simulink library "inp"  (R2021b)
settings: Solver=VariableStepAuto  StartTime=0.0  StopTime=10.0  RelTol=1e-3
undefined symbols (not defined in the file): C_TASK_5MS_S, FALSE, KINP_AcoreReadyToSlp_flg_ovrdflg, KINP_AcoreReadyToSlp_flg_ovrdval, KINP_AllowMovThd_OTA_enum_ovrdflg, KINP_AllowMovThd_OTA_enum_ovrdval, KINP_APSAngleTarget_Deg_ovrdflg, KINP_APSAngleTarget_Deg_ovrdval, KINP_APSDecReq_mps2_ovrdflg, KINP_APSDecReq_mps2_ovrdval, KINP_APSDecReqA_flg_ovrdflg, KINP_APSDecReqA_flg_ovrdval, KINP_APSDFLL_cm_ovrdflg, KINP_APSDFLL_cm_ovrdval, KINP_APSDFLR_cm_ovrdflg, KINP_APSDFLR_cm_ovrdval, KINP_APSDRLL_cm_ovrdflg, KINP_APSDRLL_cm_ovrdval, KINP_APSDRLR_cm_ovrdflg, KINP_APSDRLR_cm_ovrdval, KINP_APSExitCondition_enum_ovrdflg, KINP_APSExitCondition_enum_ovrdval, KINP_APSHWVer_enum_ovrdflg, KINP_APSHWVer_enum_ovrdval, KINP_APSProgressPCT_pct_ovrdflg, KINP_APSProgressPCT_pct_ovrdval, KINP_APSPwrReq_enum_ovrdflg, KINP_APSPwrReq_enum_ovrdval, KINP_APSReq_enum_ovrdflg, KINP_APSReq_enum_ovrdval, KINP_APSRQDisplay_enum_ovrdflg, KINP_APSRQDisplay_enum_ovrdval, KINP_APSRqEPASCtrl_flg_ovrdflg, KINP_APSRqEPASCtrl_flg_ovrdval, KINP_APSShiftPosnReq_enum_ovrdval, KINP_APSShiftPosnReq_enum_ovrflg, KINP_APSSpeedCMD_kph_ovrdval, KINP_APSSpeedCMD_kph_ovrflg, KINP_APSStaSystem_enum_ovrdflg, KINP_APSStaSystem_enum_ovrdval, KINP_APSSWVer_enum_ovrdflg, KINP_APSSWVer_enum_ovrdval, KINP_APSVMCReqA_flg_ovrdval, KINP_APSVMCReqA_flg_ovrflg, KINP_APSVRqEPASCtrl_flg_ovrdflg, KINP_APSVRqEPASCtrl_flg_ovrdval, KINP_AuxBattVolmV_mV_ovrdflg, KINP_AuxBattVolmV_mV_ovrdval, KINP_BTConnectSta_enum_ovrdflg, KINP_BTConnectSta_enum_ovrdval, KINP_CAASSta_enum_ovrdflg, KINP_CAASSta_enum_ovrdval, KINP_CAASVMCReqA_flg_ovrdval, KINP_CAASVMCReqA_flg_ovrflg, KINP_CAN1BusOff_flg_ovrdflg, KINP_CAN1BusOff_flg_ovrdval, KINP_CAN2BusOff_flg_ovrdflg, KINP_CAN2BusOff_flg_ovrdval, KINP_CAN3BusOff_flg_ovrdflg, KINP_CAN3BusOff_flg_ovrdval ... (+222)
libraries: FVT_lib x1035, hcu_lib x1
(part 33 of 33)

== system inp/INP/CAN6/SignalCheck/FCM2 ==
  BHAL_outputs : Inport
  inp_CanValid_bus : Inport  Port=2
  ADBVehDst1Val : FVT_lib/inp/can_signal_template  SystemSampleTime=-1  VariantActivationTime=update diagram  Latency=0  AutoFrameSizeCalculation=off
      link override defval: Value=KINP_ADBVehDst1Val_enum_defval
      link override ovrdflg: Value=KINP_ADBVehDst1Val_enum_ovrdflg
      link override ovrdval: Value=KINP_ADBVehDst1Val_enum_ovrdval
  FCM2CSErr : FVT_lib/inp/can_signal_template  SystemSampleTime=-1  VariantActivationTime=update diagram  Latency=0  AutoFrameSizeCalculation=off
      link override defval: Value=KINP_FCM2CSErr_flg_defval
      link override ovrdflg: Value=KINP_FCM2CSErr_flg_ovrdflg
      link override ovrdval: Value=KINP_FCM2CSErr_flg_ovrdval
  FCM2RCErr : FVT_lib/inp/can_signal_template  SystemSampleTime=-1  VariantActivationTime=update diagram  Latency=0  AutoFrameSizeCalculation=off
      link override defval: Value=KINP_FCM2RCErr_flg_defval
      link override ovrdflg: Value=KINP_FCM2RCErr_flg_ovrdflg
      link override ovrdval: Value=KINP_FCM2RCErr_flg_ovrdval
  Terminator_1 : Terminator
  Terminator_2 : Terminator
  Terminator_3 : Terminator
  True_VHAL_ADBVehDst1Val_enum : Constant  Value=TRUE  OutDataTypeStr=boolean
  True_VHAL_FCM2CSErr_flg : Constant  Value=TRUE  OutDataTypeStr=boolean
  True_VHAL_FCM2RCErr_flg : Constant  Value=TRUE  OutDataTypeStr=boolean
  slr1_1 : BusSelector  OutputSignals=VINP_CANMsgValidFCM2_flg
  slr1_2 : BusSelector  OutputSignals=VINP_CANMsgValidFCM2_flg
  slr1_3 : BusSelector  OutputSignals=VINP_CANMsgValidFCM2_flg
  slr_VHAL_ADBVehDst1Val_enum : BusSelector  OutputSignals=VHAL_ADBVehDst1Val_enum
  slr_VHAL_FCM2CSErr_flg : BusSelector  OutputSignals=VHAL_FCM2CSErr_flg
  slr_VHAL_FCM2RCErr_flg : BusSelector  OutputSignals=VHAL_FCM2RCErr_flg
  VINP_FCM2CSErr_flg : Outport
  VINP_FCM2RCErr_flg : Outport  Port=2
  VINP_ADBVehDst1Val_enum : Outport  Port=3
  wires:
  BHAL_outputs/1 -> [BHAL_outputs]
  inp_CanValid_bus/1 -> [inp_CanValid_bus]
  [BHAL_outputs] -> slr_VHAL_FCM2CSErr_flg/1
  slr_VHAL_FCM2CSErr_flg/1 -> FCM2CSErr/1  "<VHAL_FCM2CSErr_flg>"
  True_VHAL_FCM2CSErr_flg/1 -> FCM2CSErr/2
  [inp_CanValid_bus] -> slr1_1/1
  slr1_1/1 -> FCM2CSErr/3  "<VINP_CANMsgValidFCM2_flg>"
  FCM2CSErr/1 -> VINP_FCM2CSErr_flg/1  "VINP_FCM2CSErr_flg"
  FCM2CSErr/2 -> Terminator_1/1
  [BHAL_outputs] -> slr_VHAL_FCM2RCErr_flg/1
  slr_VHAL_FCM2RCErr_flg/1 -> FCM2RCErr/1  "<VHAL_FCM2RCErr_flg>"
  True_VHAL_FCM2RCErr_flg/1 -> FCM2RCErr/2
  [inp_CanValid_bus] -> slr1_2/1
  slr1_2/1 -> FCM2RCErr/3  "<VINP_CANMsgValidFCM2_flg>"
  FCM2RCErr/1 -> VINP_FCM2RCErr_flg/1  "VINP_FCM2RCErr_flg"
  FCM2RCErr/2 -> Terminator_2/1
  [BHAL_outputs] -> slr_VHAL_ADBVehDst1Val_enum/1
  slr_VHAL_ADBVehDst1Val_enum/1 -> ADBVehDst1Val/1  "<VHAL_ADBVehDst1Val_enum>"
  True_VHAL_ADBVehDst1Val_enum/1 -> ADBVehDst1Val/2
  [inp_CanValid_bus] -> slr1_3/1
  slr1_3/1 -> ADBVehDst1Val/3  "<VINP_CANMsgValidFCM2_flg>"
  ADBVehDst1Val/1 -> VINP_ADBVehDst1Val_enum/1  "VINP_ADBVehDst1Val_enum"
  ADBVehDst1Val/2 -> Terminator_3/1

== system inp/INP/CAN6/SignalCheck/FCM3 ==
  BHAL_outputs : Inport
  inp_CanValid_bus : Inport  Port=2
  MELaneCurvDervLt : FVT_lib/inp/can_signal_template  SystemSampleTime=-1  VariantActivationTime=update diagram  Latency=0  AutoFrameSizeCalculation=off
      link override defval: Value=KINP_MELaneCurvDervLt_raw32_defval
      link override ovrdflg: Value=KINP_MELaneCurvDervLt_raw32_ovrdflg
      link override ovrdval: Value=KINP_MELaneCurvDervLt_raw32_ovrdval
  MELaneCurvDervLt2 : FVT_lib/inp/can_signal_template  SystemSampleTime=-1  VariantActivationTime=update diagram  Latency=0  AutoFrameSizeCalculation=off
      link override defval: Value=KINP_MELaneCurvDervLt2_raw32_defval
      link override ovrdflg: Value=KINP_MELaneCurvDervLt2_raw32_ovrdflg
      link override ovrdval: Value=KINP_MELaneCurvDervLt2_raw32_ovrdval
  MELaneCurvDervRt : FVT_lib/inp/can_signal_template  SystemSampleTime=-1  VariantActivationTime=update diagram  Latency=0  AutoFrameSizeCalculation=off
      link override defval: Value=KINP_MELaneCurvDervRt_raw32_defval
      link override ovrdflg: Value=KINP_MELaneCurvDervRt_raw32_ovrdflg
      link override ovrdval: Value=KINP_MELaneCurvDervRt_raw32_ovrdval
  MELaneCurvDervRt2 : FVT_lib/inp/can_signal_template  SystemSampleTime=-1  VariantActivationTime=update diagram  Latency=0  AutoFrameSizeCalculation=off
      link override defval: Value=KINP_MELaneCurvDervRt2_raw32_defval
      link override ovrdflg: Value=KINP_MELaneCurvDervRt2_raw32_ovrdflg
      link override ovrdval: Value=KINP_MELaneCurvDervRt2_raw32_ovrdval
  MELaneCurvLt : FVT_lib/inp/can_signal_template  SystemSampleTime=-1  VariantActivationTime=update diagram  Latency=0  AutoFrameSizeCalculation=off
      link override defval: Value=KINP_MELaneCurvLt_raw32_defval
      link override ovrdflg: Value=KINP_MELaneCurvLt_raw32_ovrdflg
      link override ovrdval: Value=KINP_MELaneCurvLt_raw32_ovrdval
  MELaneCurvLt2 : FVT_lib/inp/can_signal_template  SystemSampleTime=-1  VariantActivationTime=update diagram  Latency=0  AutoFrameSizeCalculation=off
      link override defval: Value=KINP_MELaneCurvLt2_raw32_defval
      link override ovrdflg: Value=KINP_MELaneCurvLt2_raw32_ovrdflg
      link override ovrdval: Value=KINP_MELaneCurvLt2_raw32_ovrdval
  MELaneCurvRt : FVT_lib/inp/can_signal_template  SystemSampleTime=-1  VariantActivationTime=update diagram  Latency=0  AutoFrameSizeCalculation=off
      link override defval: Value=KINP_MELaneCurvRt_raw32_defval
      link override ovrdflg: Value=KINP_MELaneCurvRt_raw32_ovrdflg
      link override ovrdval: Value=KINP_MELaneCurvRt_raw32_ovrdval
  MELaneCurvRt2 : FVT_lib/inp/can_signal_template  SystemSampleTime=-1  VariantActivationTime=update diagram  Latency=0  AutoFrameSizeCalculation=off
      link override defval: Value=KINP_MELaneCurvRt2_raw32_defval
      link override ovrdflg: Value=KINP_MELaneCurvRt2_raw32_ovrdflg
      link override ovrdval: Value=KINP_MELaneCurvRt2_raw32_ovrdval
  MELaneHeadAngLt : FVT_lib/inp/can_signal_template  SystemSampleTime=-1  VariantActivationTime=update diagram  Latency=0  AutoFrameSizeCalculation=off
      link override defval: Value=KINP_MELaneHeadAngLt_radians_defval
      link override ovrdflg: Value=KINP_MELaneHeadAngLt_radians_ovrdflg
      link override ovrdval: Value=KINP_MELaneHeadAngLt_radians_ovrdval
  MELaneHeadAngLt2 : FVT_lib/inp/can_signal_template  SystemSampleTime=-1  VariantActivationTime=update diagram  Latency=0  AutoFrameSizeCalculation=off
      link override defval: Value=KINP_MELaneHeadAngLt2_radians_defval
      link override ovrdflg: Value=KINP_MELaneHeadAngLt2_radians_ovrdflg
      link override ovrdval: Value=KINP_MELaneHeadAngLt2_radians_ovrdval
  MELaneHeadAngRt : FVT_lib/inp/can_signal_template  SystemSampleTime=-1  VariantActivationTime=update diagram  Latency=0  AutoFrameSizeCalculation=off
      link override defval: Value=KINP_MELaneHeadAngRt_radians_defval
      link override ovrdflg: Value=KINP_MELaneHeadAngRt_radians_ovrdflg
      link override ovrdval: Value=KINP_MELaneHeadAngRt_radians_ovrdval
  MELaneHeadAngRt2 : FVT_lib/inp/can_signal_template  SystemSampleTime=-1  VariantActivationTime=update diagram  Latency=0  AutoFrameSizeCalculation=off
      link override defval: Value=KINP_MELaneHeadAngRt2_radians_defval
      link override ovrdflg: Value=KINP_MELaneHeadAngRt2_radians_ovrdflg
      link override ovrdval: Value=KINP_MELaneHeadAngRt2_radians_ovrdval
  MELanePosLt : FVT_lib/inp/can_signal_template  SystemSampleTime=-1  VariantActivationTime=update diagram  Latency=0  AutoFrameSizeCalculation=off
      link override defval: Value=KINP_MELanePosLt_m_defval
      link override ovrdflg: Value=KINP_MELanePosLt_m_ovrdflg
      link override ovrdval: Value=KINP_MELanePosLt_m_ovrdval
  MELanePosLt2 : FVT_lib/inp/can_signal_template  SystemSampleTime=-1  VariantActivationTime=update diagram  Latency=0  AutoFrameSizeCalculation=off
      link override defval: Value=KINP_MELanePosLt2_m_defval
      link override ovrdflg: Value=KINP_MELanePosLt2_m_ovrdflg
      link override ovrdval: Value=KINP_MELanePosLt2_m_ovrdval
  MELanePosRt : FVT_lib/inp/can_signal_template  SystemSampleTime=-1  VariantActivationTime=update diagram  Latency=0  AutoFrameSizeCalculation=off
      link override defval: Value=KINP_MELanePosRt_m_defval
      link override ovrdflg: Value=KINP_MELanePosRt_m_ovrdflg
      link override ovrdval: Value=KINP_MELanePosRt_m_ovrdval
  MELanePosRt2 : FVT_lib/inp/can_signal_template  SystemSampleTime=-1  VariantActivationTime=update diagram  Latency=0  AutoFrameSizeCalculation=off
      link override defval: Value=KINP_MELanePosRt2_m_defval
      link override ovrdflg: Value=KINP_MELanePosRt2_m_ovrdflg
      link override ovrdval: Value=KINP_MELanePosRt2_m_ovrdval
  Terminator_{1..16} (16 alike) : Terminator
  True_VHAL_MELaneCurvDervLt2_raw32 : Constant  Value=TRUE  OutDataTypeStr=boolean
  True_VHAL_MELaneCurvDervLt_raw32 : Constant  Value=TRUE  OutDataTypeStr=boolean
  True_VHAL_MELaneCurvDervRt2_raw32 : Constant  Value=TRUE  OutDataTypeStr=boolean
  True_VHAL_MELaneCurvDervRt_raw32 : Constant  Value=TRUE  OutDataTypeStr=boolean
  True_VHAL_MELaneCurvLt2_raw32 : Constant  Value=TRUE  OutDataTypeStr=boolean
  True_VHAL_MELaneCurvLt_raw32 : Constant  Value=TRUE  OutDataTypeStr=boolean
  True_VHAL_MELaneCurvRt2_raw32 : Constant  Value=TRUE  OutDataTypeStr=boolean
  True_VHAL_MELaneCurvRt_raw32 : Constant  Value=TRUE  OutDataTypeStr=boolean
  True_VHAL_MELaneHeadAngLt2_radians : Constant  Value=TRUE  OutDataTypeStr=boolean
  True_VHAL_MELaneHeadAngLt_radians : Constant  Value=TRUE  OutDataTypeStr=boolean
  True_VHAL_MELaneHeadAngRt2_radians : Constant  Value=TRUE  OutDataTypeStr=boolean
  True_VHAL_MELaneHeadAngRt_radians : Constant  Value=TRUE  OutDataTypeStr=boolean
  True_VHAL_MELanePosLt2_m : Constant  Value=TRUE  OutDataTypeStr=boolean
  True_VHAL_MELanePosLt_m : Constant  Value=TRUE  OutDataTypeStr=boolean
  True_VHAL_MELanePosRt2_m : Constant  Value=TRUE  OutDataTypeStr=boolean
  True_VHAL_MELanePosRt_m : Constant  Value=TRUE  OutDataTypeStr=boolean
  slr1_{1..16} (16 alike) : BusSelector  OutputSignals=VINP_CANMsgValidFCM3_flg
  slr_VHAL_MELaneCurvDervLt2_raw32 : BusSelector  OutputSignals=VHAL_MELaneCurvDervLt2_raw32
  slr_VHAL_MELaneCurvDervLt_raw32 : BusSelector  OutputSignals=VHAL_MELaneCurvDervLt_raw32
  slr_VHAL_MELaneCurvDervRt2_raw32 : BusSelector  OutputSignals=VHAL_MELaneCurvDervRt2_raw32
  slr_VHAL_MELaneCurvDervRt_raw32 : BusSelector  OutputSignals=VHAL_MELaneCurvDervRt_raw32
  slr_VHAL_MELaneCurvLt2_raw32 : BusSelector  OutputSignals=VHAL_MELaneCurvLt2_raw32
  slr_VHAL_MELaneCurvLt_raw32 : BusSelector  OutputSignals=VHAL_MELaneCurvLt_raw32
  slr_VHAL_MELaneCurvRt2_raw32 : BusSelector  OutputSignals=VHAL_MELaneCurvRt2_raw32
  slr_VHAL_MELaneCurvRt_raw32 : BusSelector  OutputSignals=VHAL_MELaneCurvRt_raw32
  slr_VHAL_MELaneHeadAngLt2_radians : BusSelector  OutputSignals=VHAL_MELaneHeadAngLt2_radians
  slr_VHAL_MELaneHeadAngLt_radians : BusSelector  OutputSignals=VHAL_MELaneHeadAngLt_radians
  slr_VHAL_MELaneHeadAngRt2_radians : BusSelector  OutputSignals=VHAL_MELaneHeadAngRt2_radians
  slr_VHAL_MELaneHeadAngRt_radians : BusSelector  OutputSignals=VHAL_MELaneHeadAngRt_radians
  slr_VHAL_MELanePosLt2_m : BusSelector  OutputSignals=VHAL_MELanePosLt2_m
  slr_VHAL_MELanePosLt_m : BusSelector  OutputSignals=VHAL_MELanePosLt_m
  slr_VHAL_MELanePosRt2_m : BusSelector  OutputSignals=VHAL_MELanePosRt2_m
  slr_VHAL_MELanePosRt_m : BusSelector  OutputSignals=VHAL_MELanePosRt_m
  VINP_MELaneCurvDervLt_raw32 : Outport
  VINP_MELaneCurvDervLt2_raw32 : Outport  Port=2
  VINP_MELaneCurvDervRt_raw32 : Outport  Port=3
  VINP_MELaneCurvDervRt2_raw32 : Outport  Port=4
  VINP_MELaneCurvLt_raw32 : Outport  Port=5
  VINP_MELaneCurvLt2_raw32 : Outport  Port=6
  VINP_MELaneCurvRt_raw32 : Outport  Port=7
  VINP_MELaneCurvRt2_raw32 : Outport  Port=8
  VINP_MELaneHeadAngLt_radians : Outport  Port=9
  VINP_MELaneHeadAngLt2_radians : Outport  Port=10
  VINP_MELaneHeadAngRt_radians : Outport  Port=11
  VINP_MELaneHeadAngRt2_radians : Outport  Port=12
  VINP_MELanePosLt_m : Outport  Port=13
  VINP_MELanePosLt2_m : Outport  Port=14
  VINP_MELanePosRt_m : Outport  Port=15
  VINP_MELanePosRt2_m : Outport  Port=16
  wires:
  BHAL_outputs/1 -> [BHAL_outputs]
  inp_CanValid_bus/1 -> [inp_CanValid_bus]
  [BHAL_outputs] -> slr_VHAL_MELaneCurvDervLt_raw32/1
  slr_VHAL_MELaneCurvDervLt_raw32/1 -> MELaneCurvDervLt/1  "<VHAL_MELaneCurvDervLt_raw32>"
  True_VHAL_MELaneCurvDervLt_raw32/1 -> MELaneCurvDervLt/2
  [inp_CanValid_bus] -> slr1_1/1
  slr1_1/1 -> MELaneCurvDervLt/3  "<VINP_CANMsgValidFCM3_flg>"
  MELaneCurvDervLt/1 -> VINP_MELaneCurvDervLt_raw32/1  "VINP_MELaneCurvDervLt_raw32"
  MELaneCurvDervLt/2 -> Terminator_1/1
  [BHAL_outputs] -> slr_VHAL_MELaneCurvDervLt2_raw32/1
  slr_VHAL_MELaneCurvDervLt2_raw32/1 -> MELaneCurvDervLt2/1  "<VHAL_MELaneCurvDervLt2_raw32>"
  True_VHAL_MELaneCurvDervLt2_raw32/1 -> MELaneCurvDervLt2/2
  [inp_CanValid_bus] -> slr1_2/1
  slr1_2/1 -> MELaneCurvDervLt2/3  "<VINP_CANMsgValidFCM3_flg>"
  MELaneCurvDervLt2/1 -> VINP_MELaneCurvDervLt2_raw32/1  "VINP_MELaneCurvDervLt2_raw32"
  MELaneCurvDervLt2/2 -> Terminator_2/1
  [BHAL_outputs] -> slr_VHAL_MELaneCurvDervRt_raw32/1
  slr_VHAL_MELaneCurvDervRt_raw32/1 -> MELaneCurvDervRt/1  "<VHAL_MELaneCurvDervRt_raw32>"
  True_VHAL_MELaneCurvDervRt_raw32/1 -> MELaneCurvDervRt/2
  [inp_CanValid_bus] -> slr1_3/1
  slr1_3/1 -> MELaneCurvDervRt/3  "<VINP_CANMsgValidFCM3_flg>"
  MELaneCurvDervRt/1 -> VINP_MELaneCurvDervRt_raw32/1  "VINP_MELaneCurvDervRt_raw32"
  MELaneCurvDervRt/2 -> Terminator_3/1
  [BHAL_outputs] -> slr_VHAL_MELaneCurvDervRt2_raw32/1
  slr_VHAL_MELaneCurvDervRt2_raw32/1 -> MELaneCurvDervRt2/1  "<VHAL_MELaneCurvDervRt2_raw32>"
  True_VHAL_MELaneCurvDervRt2_raw32/1 -> MELaneCurvDervRt2/2
  [inp_CanValid_bus] -> slr1_4/1
  slr1_4/1 -> MELaneCurvDervRt2/3  "<VINP_CANMsgValidFCM3_flg>"
  MELaneCurvDervRt2/1 -> VINP_MELaneCurvDervRt2_raw32/1  "VINP_MELaneCurvDervRt2_raw32"
  MELaneCurvDervRt2/2 -> Terminator_4/1
  [BHAL_outputs] -> slr_VHAL_MELaneCurvLt_raw32/1
  slr_VHAL_MELaneCurvLt_raw32/1 -> MELaneCurvLt/1  "<VHAL_MELaneCurvLt_raw32>"
  True_VHAL_MELaneCurvLt_raw32/1 -> MELaneCurvLt/2
  [inp_CanValid_bus] -> slr1_5/1
  slr1_5/1 -> MELaneCurvLt/3  "<VINP_CANMsgValidFCM3_flg>"
  MELaneCurvLt/1 -> VINP_MELaneCurvLt_raw32/1  "VINP_MELaneCurvLt_raw32"
  MELaneCurvLt/2 -> Terminator_5/1
  [BHAL_outputs] -> slr_VHAL_MELaneCurvLt2_raw32/1
  slr_VHAL_MELaneCurvLt2_raw32/1 -> MELaneCurvLt2/1  "<VHAL_MELaneCurvLt2_raw32>"
  True_VHAL_MELaneCurvLt2_raw32/1 -> MELaneCurvLt2/2
  [inp_CanValid_bus] -> slr1_6/1
  slr1_6/1 -> MELaneCurvLt2/3  "<VINP_CANMsgValidFCM3_flg>"
  MELaneCurvLt2/1 -> VINP_MELaneCurvLt2_raw32/1  "VINP_MELaneCurvLt2_raw32"
  MELaneCurvLt2/2 -> Terminator_6/1
  [BHAL_outputs] -> slr_VHAL_MELaneCurvRt_raw32/1
  slr_VHAL_MELaneCurvRt_raw32/1 -> MELaneCurvRt/1  "<VHAL_MELaneCurvRt_raw32>"
  True_VHAL_MELaneCurvRt_raw32/1 -> MELaneCurvRt/2
  [inp_CanValid_bus] -> slr1_7/1
  slr1_7/1 -> MELaneCurvRt/3  "<VINP_CANMsgValidFCM3_flg>"
  MELaneCurvRt/1 -> VINP_MELaneCurvRt_raw32/1  "VINP_MELaneCurvRt_raw32"
  MELaneCurvRt/2 -> Terminator_7/1
  [BHAL_outputs] -> slr_VHAL_MELaneCurvRt2_raw32/1
  slr_VHAL_MELaneCurvRt2_raw32/1 -> MELaneCurvRt2/1  "<VHAL_MELaneCurvRt2_raw32>"
  True_VHAL_MELaneCurvRt2_raw32/1 -> MELaneCurvRt2/2
  [inp_CanValid_bus] -> slr1_8/1
  slr1_8/1 -> MELaneCurvRt2/3  "<VINP_CANMsgValidFCM3_flg>"
  MELaneCurvRt2/1 -> VINP_MELaneCurvRt2_raw32/1  "VINP_MELaneCurvRt2_raw32"
  MELaneCurvRt2/2 -> Terminator_8/1
  [BHAL_outputs] -> slr_VHAL_MELaneHeadAngLt_radians/1
  slr_VHAL_MELaneHeadAngLt_radians/1 -> MELaneHeadAngLt/1  "<VHAL_MELaneHeadAngLt_radians>"
  True_VHAL_MELaneHeadAngLt_radians/1 -> MELaneHeadAngLt/2
  [inp_CanValid_bus] -> slr1_9/1
  slr1_9/1 -> MELaneHeadAngLt/3  "<VINP_CANMsgValidFCM3_flg>"
  MELaneHeadAngLt/1 -> VINP_MELaneHeadAngLt_radians/1  "VINP_MELaneHeadAngLt_radians"
  MELaneHeadAngLt/2 -> Terminator_9/1
  [BHAL_outputs] -> slr_VHAL_MELaneHeadAngLt2_radians/1
  slr_VHAL_MELaneHeadAngLt2_radians/1 -> MELaneHeadAngLt2/1  "<VHAL_MELaneHeadAngLt2_radians>"
  True_VHAL_MELaneHeadAngLt2_radians/1 -> MELaneHeadAngLt2/2
  [inp_CanValid_bus] -> slr1_10/1
  slr1_10/1 -> MELaneHeadAngLt2/3  "<VINP_CANMsgValidFCM3_flg>"
  MELaneHeadAngLt2/1 -> VINP_MELaneHeadAngLt2_radians/1  "VINP_MELaneHeadAngLt2_radians"
  MELaneHeadAngLt2/2 -> Terminator_10/1
  [BHAL_outputs] -> slr_VHAL_MELaneHeadAngRt_radians/1
  slr_VHAL_MELaneHeadAngRt_radians/1 -> MELaneHeadAngRt/1  "<VHAL_MELaneHeadAngRt_radians>"
  True_VHAL_MELaneHeadAngRt_radians/1 -> MELaneHeadAngRt/2
  [inp_CanValid_bus] -> slr1_11/1
  slr1_11/1 -> MELaneHeadAngRt/3  "<VINP_CANMsgValidFCM3_flg>"
  MELaneHeadAngRt/1 -> VINP_MELaneHeadAngRt_radians/1  "VINP_MELaneHeadAngRt_radians"
  MELaneHeadAngRt/2 -> Terminator_11/1
  [BHAL_outputs] -> slr_VHAL_MELaneHeadAngRt2_radians/1
  slr_VHAL_MELaneHeadAngRt2_radians/1 -> MELaneHeadAngRt2/1  "<VHAL_MELaneHeadAngRt2_radians>"
  True_VHAL_MELaneHeadAngRt2_radians/1 -> MELaneHeadAngRt2/2
  [inp_CanValid_bus] -> slr1_12/1
  slr1_12/1 -> MELaneHeadAngRt2/3  "<VINP_CANMsgValidFCM3_flg>"
  MELaneHeadAngRt2/1 -> VINP_MELaneHeadAngRt2_radians/1  "VINP_MELaneHeadAngRt2_radians"
  MELaneHeadAngRt2/2 -> Terminator_12/1
  [BHAL_outputs] -> slr_VHAL_MELanePosLt_m/1
  slr_VHAL_MELanePosLt_m/1 -> MELanePosLt/1  "<VHAL_MELanePosLt_m>"
  True_VHAL_MELanePosLt_m/1 -> MELanePosLt/2
  [inp_CanValid_bus] -> slr1_13/1
  slr1_13/1 -> MELanePosLt/3  "<VINP_CANMsgValidFCM3_flg>"
  MELanePosLt/1 -> VINP_MELanePosLt_m/1  "VINP_MELanePosLt_m"
  MELanePosLt/2 -> Terminator_13/1
  [BHAL_outputs] -> slr_VHAL_MELanePosLt2_m/1
  slr_VHAL_MELanePosLt2_m/1 -> MELanePosLt2/1  "<VHAL_MELanePosLt2_m>"
  True_VHAL_MELanePosLt2_m/1 -> MELanePosLt2/2
  [inp_CanValid_bus] -> slr1_14/1
  slr1_14/1 -> MELanePosLt2/3  "<VINP_CANMsgValidFCM3_flg>"
  MELanePosLt2/1 -> VINP_MELanePosLt2_m/1  "VINP_MELanePosLt2_m"
  MELanePosLt2/2 -> Terminator_14/1
  [BHAL_outputs] -> slr_VHAL_MELanePosRt_m/1
  slr_VHAL_MELanePosRt_m/1 -> MELanePosRt/1  "<VHAL_MELanePosRt_m>"
  True_VHAL_MELanePosRt_m/1 -> MELanePosRt/2
  [inp_CanValid_bus] -> slr1_15/1
  slr1_15/1 -> MELanePosRt/3  "<VINP_CANMsgValidFCM3_flg>"
  MELanePosRt/1 -> VINP_MELanePosRt_m/1  "VINP_MELanePosRt_m"
  MELanePosRt/2 -> Terminator_15/1
  [BHAL_outputs] -> slr_VHAL_MELanePosRt2_m/1
  slr_VHAL_MELanePosRt2_m/1 -> MELanePosRt2/1  "<VHAL_MELanePosRt2_m>"
  True_VHAL_MELanePosRt2_m/1 -> MELanePosRt2/2
  [inp_CanValid_bus] -> slr1_16/1
  slr1_16/1 -> MELanePosRt2/3  "<VINP_CANMsgValidFCM3_flg>"
  MELanePosRt2/1 -> VINP_MELanePosRt2_m/1  "VINP_MELanePosRt2_m"
  MELanePosRt2/2 -> Terminator_16/1

== system inp/INP/CAN6/SignalCheck/FCM4 ==
  BHAL_outputs : Inport
  inp_CanValid_bus : Inport  Port=2
  ADASAngCtrlTqWeightGain : FVT_lib/inp/can_signal_template  SystemSampleTime=-1  VariantActivationTime=update diagram  Latency=0  AutoFrameSizeCalculation=off
      link override defval: Value=KINP_ADASAngCtrlTqWeightGain_pct_defval
      link override ovrdflg: Value=KINP_ADASAngCtrlTqWeightGain_pct_ovrdflg
      link override ovrdval: Value=KINP_ADASAngCtrlTqWeightGain_pct_ovrdval
  ADASDesStrWhlAngCtrlCmd : FVT_lib/inp/can_signal_template  SystemSampleTime=-1  VariantActivationTime=update diagram  Latency=0  AutoFrameSizeCalculation=off
      link override defval: Value=KINP_ADASDesStrWhlAngCtrlCmd_Deg_defval
      link override ovrdflg: Value=KINP_ADASDesStrWhlAngCtrlCmd_Deg_ovrdflg
      link override ovrdval: Value=KINP_ADASDesStrWhlAngCtrlCmd_Deg_ovrdval
  ADASDrvInputTqBoostAct : FVT_lib/inp/can_signal_template  SystemSampleTime=-1  VariantActivationTime=update diagram  Latency=0  AutoFrameSizeCalculation=off
      link override defval: Value=KINP_ADASDrvInputTqBoostAct_flg_defval
      link override ovrdflg: Value=KINP_ADASDrvInputTqBoostAct_flg_ovrdflg
      link override ovrdval: Value=KINP_ADASDrvInputTqBoostAct_flg_ovrdval
  ADASDrvInputTqBoostGain : FVT_lib/inp/can_signal_template  SystemSampleTime=-1  VariantActivationTime=update diagram  Latency=0  AutoFrameSizeCalculation=off
      link override defval: Value=KINP_ADASDrvInputTqBoostGain_pct_defval
      link override ovrdflg: Value=KINP_ADASDrvInputTqBoostGain_pct_ovrdflg
      link override ovrdval: Value=KINP_ADASDrvInputTqBoostGain_pct_ovrdval
  ADASMaxAngCtrlOutTqLimit : FVT_lib/inp/can_signal_template  SystemSampleTime=-1  VariantActivationTime=update diagram  Latency=0  AutoFrameSizeCalculation=off
      link override defval: Value=KINP_ADASMaxAngCtrlOutTqLimit_Nm_defval
      link override ovrdflg: Value=KINP_ADASMaxAngCtrlOutTqLimit_Nm_ovrdflg
      link override ovrdval: Value=KINP_ADASMaxAngCtrlOutTqLimit_Nm_ovrdval
  ADASStrWhlAngCtrlStatus : FVT_lib/inp/can_signal_template  SystemSampleTime=-1  VariantActivationTime=update diagram  Latency=0  AutoFrameSizeCalculation=off
      link override defval: Value=KINP_ADASStrWhlAngCtrlStatus_flg_defval
      link override ovrdflg: Value=KINP_ADASStrWhlAngCtrlStatus_flg_ovrdflg
      link override ovrdval: Value=KINP_ADASStrWhlAngCtrlStatus_flg_ovrdval
  FCM4CSErr : FVT_lib/inp/can_signal_template  SystemSampleTime=-1  VariantActivationTime=update diagram  Latency=0  AutoFrameSizeCalculation=off
      link override defval: Value=KINP_FCM4CSErr_flg_defval
      link override ovrdflg: Value=KINP_FCM4CSErr_flg_ovrdflg
      link override ovrdval: Value=KINP_FCM4CSErr_flg_ovrdval
  FCM4RCErr : FVT_lib/inp/can_signal_template  SystemSampleTime=-1  VariantActivationTime=update diagram  Latency=0  AutoFrameSizeCalculation=off
      link override defval: Value=KINP_FCM4RCErr_flg_defval
      link override ovrdflg: Value=KINP_FCM4RCErr_flg_ovrdflg
      link override ovrdval: Value=KINP_FCM4RCErr_flg_ovrdval
  Terminator_{1..8} (8 alike) : Terminator
  True_VHAL_ADASAngCtrlTqWeightGain_pct : Constant  Value=TRUE  OutDataTypeStr=boolean
  True_VHAL_ADASDesStrWhlAngCtrlCmd_Deg : Constant  Value=TRUE  OutDataTypeStr=boolean
  True_VHAL_ADASDrvInputTqBoostAct_flg : Constant  Value=TRUE  OutDataTypeStr=boolean
  True_VHAL_ADASDrvInputTqBoostGain_pct : Constant  Value=TRUE  OutDataTypeStr=boolean
  True_VHAL_ADASMaxAngCtrlOutTqLimit_Nm : Constant  Value=TRUE  OutDataTypeStr=boolean
  True_VHAL_ADASStrWhlAngCtrlStatus_flg : Constant  Value=TRUE  OutDataTypeStr=boolean
  True_VHAL_FCM4CSErr_flg : Constant  Value=TRUE  OutDataTypeStr=boolean
  True_VHAL_FCM4RCErr_flg : Constant  Value=TRUE  OutDataTypeStr=boolean
  slr1_{1..8} (8 alike) : BusSelector  OutputSignals=VINP_CANMsgValidFCM4_flg
  slr_VHAL_ADASAngCtrlTqWeightGain_pct : BusSelector  OutputSignals=VHAL_ADASAngCtrlTqWeightGain_pct
  slr_VHAL_ADASDesStrWhlAngCtrlCmd_Deg : BusSelector  OutputSignals=VHAL_ADASDesStrWhlAngCtrlCmd_Deg
  slr_VHAL_ADASDrvInputTqBoostAct_flg : BusSelector  OutputSignals=VHAL_ADASDrvInputTqBoostAct_flg
  slr_VHAL_ADASDrvInputTqBoostGain_pct : BusSelector  OutputSignals=VHAL_ADASDrvInputTqBoostGain_pct
  slr_VHAL_ADASMaxAngCtrlOutTqLimit_Nm : BusSelector  OutputSignals=VHAL_ADASMaxAngCtrlOutTqLimit_Nm
  slr_VHAL_ADASStrWhlAngCtrlStatus_flg : BusSelector  OutputSignals=VHAL_ADASStrWhlAngCtrlStatus_flg
  slr_VHAL_FCM4CSErr_flg : BusSelector  OutputSignals=VHAL_FCM4CSErr_flg
  slr_VHAL_FCM4RCErr_flg : BusSelector  OutputSignals=VHAL_FCM4RCErr_flg
  VINP_FCM4CSErr_flg : Outport
  VINP_FCM4RCErr_flg : Outport  Port=2
  VINP_ADASAngCtrlTqWeightGain_pct : Outport  Port=3
  VINP_ADASDesStrWhlAngCtrlCmd_Deg : Outport  Port=4
  VINP_ADASDrvInputTqBoostAct_flg : Outport  Port=5
  VINP_ADASDrvInputTqBoostGain_pct : Outport  Port=6
  VINP_ADASMaxAngCtrlOutTqLimit_Nm : Outport  Port=7
  VINP_ADASStrWhlAngCtrlStatus_flg : Outport  Port=8
  wires:
  BHAL_outputs/1 -> [BHAL_outputs]
  inp_CanValid_bus/1 -> [inp_CanValid_bus]
  [BHAL_outputs] -> slr_VHAL_FCM4CSErr_flg/1
  slr_VHAL_FCM4CSErr_flg/1 -> FCM4CSErr/1  "<VHAL_FCM4CSErr_flg>"
  True_VHAL_FCM4CSErr_flg/1 -> FCM4CSErr/2
  [inp_CanValid_bus] -> slr1_1/1
  slr1_1/1 -> FCM4CSErr/3  "<VINP_CANMsgValidFCM4_flg>"
  FCM4CSErr/1 -> VINP_FCM4CSErr_flg/1  "VINP_FCM4CSErr_flg"
  FCM4CSErr/2 -> Terminator_1/1
  [BHAL_outputs] -> slr_VHAL_FCM4RCErr_flg/1
  slr_VHAL_FCM4RCErr_flg/1 -> FCM4RCErr/1  "<VHAL_FCM4RCErr_flg>"
  True_VHAL_FCM4RCErr_flg/1 -> FCM4RCErr/2
  [inp_CanValid_bus] -> slr1_2/1
  slr1_2/1 -> FCM4RCErr/3  "<VINP_CANMsgValidFCM4_flg>"
  FCM4RCErr/1 -> VINP_FCM4RCErr_flg/1  "VINP_FCM4RCErr_flg"
  FCM4RCErr/2 -> Terminator_2/1
  [BHAL_outputs] -> slr_VHAL_ADASAngCtrlTqWeightGain_pct/1
  slr_VHAL_ADASAngCtrlTqWeightGain_pct/1 -> ADASAngCtrlTqWeightGain/1  "<VHAL_ADASAngCtrlTqWeightGain_pct>"
  True_VHAL_ADASAngCtrlTqWeightGain_pct/1 -> ADASAngCtrlTqWeightGain/2
  [inp_CanValid_bus] -> slr1_3/1
  slr1_3/1 -> ADASAngCtrlTqWeightGain/3  "<VINP_CANMsgValidFCM4_flg>"
  ADASAngCtrlTqWeightGain/1 -> VINP_ADASAngCtrlTqWeightGain_pct/1  "VINP_ADASAngCtrlTqWeightGain_pct"
  ADASAngCtrlTqWeightGain/2 -> Terminator_3/1
  [BHAL_outputs] -> slr_VHAL_ADASDesStrWhlAngCtrlCmd_Deg/1
  slr_VHAL_ADASDesStrWhlAngCtrlCmd_Deg/1 -> ADASDesStrWhlAngCtrlCmd/1  "<VHAL_ADASDesStrWhlAngCtrlCmd_Deg>"
  True_VHAL_ADASDesStrWhlAngCtrlCmd_Deg/1 -> ADASDesStrWhlAngCtrlCmd/2
  [inp_CanValid_bus] -> slr1_4/1
  slr1_4/1 -> ADASDesStrWhlAngCtrlCmd/3  "<VINP_CANMsgValidFCM4_flg>"
  ADASDesStrWhlAngCtrlCmd/1 -> VINP_ADASDesStrWhlAngCtrlCmd_Deg/1  "VINP_ADASDesStrWhlAngCtrlCmd_Deg"
  ADASDesStrWhlAngCtrlCmd/2 -> Terminator_4/1
  [BHAL_outputs] -> slr_VHAL_ADASDrvInputTqBoostAct_flg/1
  slr_VHAL_ADASDrvInputTqBoostAct_flg/1 -> ADASDrvInputTqBoostAct/1  "<VHAL_ADASDrvInputTqBoostAct_flg>"
  True_VHAL_ADASDrvInputTqBoostAct_flg/1 -> ADASDrvInputTqBoostAct/2
  [inp_CanValid_bus] -> slr1_5/1
  slr1_5/1 -> ADASDrvInputTqBoostAct/3  "<VINP_CANMsgValidFCM4_flg>"
  ADASDrvInputTqBoostAct/1 -> VINP_ADASDrvInputTqBoostAct_flg/1  "VINP_ADASDrvInputTqBoostAct_flg"
  ADASDrvInputTqBoostAct/2 -> Terminator_5/1
  [BHAL_outputs] -> slr_VHAL_ADASDrvInputTqBoostGain_pct/1
  slr_VHAL_ADASDrvInputTqBoostGain_pct/1 -> ADASDrvInputTqBoostGain/1  "<VHAL_ADASDrvInputTqBoostGain_pct>"
  True_VHAL_ADASDrvInputTqBoostGain_pct/1 -> ADASDrvInputTqBoostGain/2
  [inp_CanValid_bus] -> slr1_6/1
  slr1_6/1 -> ADASDrvInputTqBoostGain/3  "<VINP_CANMsgValidFCM4_flg>"
  ADASDrvInputTqBoostGain/1 -> VINP_ADASDrvInputTqBoostGain_pct/1  "VINP_ADASDrvInputTqBoostGain_pct"
  ADASDrvInputTqBoostGain/2 -> Terminator_6/1
  [BHAL_outputs] -> slr_VHAL_ADASMaxAngCtrlOutTqLimit_Nm/1
  slr_VHAL_ADASMaxAngCtrlOutTqLimit_Nm/1 -> ADASMaxAngCtrlOutTqLimit/1  "<VHAL_ADASMaxAngCtrlOutTqLimit_Nm>"
  True_VHAL_ADASMaxAngCtrlOutTqLimit_Nm/1 -> ADASMaxAngCtrlOutTqLimit/2
  [inp_CanValid_bus] -> slr1_7/1
  slr1_7/1 -> ADASMaxAngCtrlOutTqLimit/3  "<VINP_CANMsgValidFCM4_flg>"
  ADASMaxAngCtrlOutTqLimit/1 -> VINP_ADASMaxAngCtrlOutTqLimit_Nm/1  "VINP_ADASMaxAngCtrlOutTqLimit_Nm"
  ADASMaxAngCtrlOutTqLimit/2 -> Terminator_7/1
  [BHAL_outputs] -> slr_VHAL_ADASStrWhlAngCtrlStatus_flg/1
  slr_VHAL_ADASStrWhlAngCtrlStatus_flg/1 -> ADASStrWhlAngCtrlStatus/1  "<VHAL_ADASStrWhlAngCtrlStatus_flg>"
  True_VHAL_ADASStrWhlAngCtrlStatus_flg/1 -> ADASStrWhlAngCtrlStatus/2
  [inp_CanValid_bus] -> slr1_8/1
  slr1_8/1 -> ADASStrWhlAngCtrlStatus/3  "<VINP_CANMsgValidFCM4_flg>"
  ADASStrWhlAngCtrlStatus/1 -> VINP_ADASStrWhlAngCtrlStatus_flg/1  "VINP_ADASStrWhlAngCtrlStatus_flg"
  ADASStrWhlAngCtrlStatus/2 -> Terminator_8/1

== system inp/INP/CAN6/SignalCheck/SRR1 ==
  BHAL_outputs : Inport
  inp_CanValid_bus : Inport  Port=2
  SRRBSDWarnL : FVT_lib/inp/can_signal_template  SystemSampleTime=-1  VariantActivationTime=update diagram  Latency=0  AutoFrameSizeCalculation=off
      link override defval: Value=KINP_SRRBSDWarnL_enum_defval
      link override ovrdflg: Value=KINP_SRRBSDWarnL_enum_ovrdflg
      link override ovrdval: Value=KINP_SRRBSDWarnL_enum_ovrdval
  SRRBSDWarnR : FVT_lib/inp/can_signal_template  SystemSampleTime=-1  VariantActivationTime=update diagram  Latency=0  AutoFrameSizeCalculation=off
      link override defval: Value=KINP_SRRBSDWarnR_enum_defval
      link override ovrdflg: Value=KINP_SRRBSDWarnR_enum_ovrdflg
      link override ovrdval: Value=KINP_SRRBSDWarnR_enum_ovrdval
  SRRODASoundL : FVT_lib/inp/can_signal_template  SystemSampleTime=-1  VariantActivationTime=update diagram  Latency=0  AutoFrameSizeCalculation=off
      link override defval: Value=KINP_SRRODASoundL_flg_defval
      link override ovrdflg: Value=KINP_SRRODASoundL_flg_ovrdflg
      link override ovrdval: Value=KINP_SRRODASoundL_flg_ovrdval
  SRRODASoundR : FVT_lib/inp/can_signal_template  SystemSampleTime=-1  VariantActivationTime=update diagram  Latency=0  AutoFrameSizeCalculation=off
      link override defval: Value=KINP_SRRODASoundR_flg_defval
      link override ovrdflg: Value=KINP_SRRODASoundR_flg_ovrdflg
      link override ovrdval: Value=KINP_SRRODASoundR_flg_ovrdval
  SRRODAWarnL : FVT_lib/inp/can_signal_template  SystemSampleTime=-1  VariantActivationTime=update diagram  Latency=0  AutoFrameSizeCalculation=off
      link override defval: Value=KINP_SRRODAWarnL_enum_defval
      link override ovrdflg: Value=KINP_SRRODAWarnL_enum_ovrdflg
      link override ovrdval: Value=KINP_SRRODAWarnL_enum_ovrdval
  SRRODAWarnR : FVT_lib/inp/can_signal_template  SystemSampleTime=-1  VariantActivationTime=update diagram  Latency=0  AutoFrameSizeCalculation=off
      link override defval: Value=KINP_SRRODAWarnR_enum_defval
      link override ovrdflg: Value=KINP_SRRODAWarnR_enum_ovrdflg
      link override ovrdval: Value=KINP_SRRODAWarnR_enum_ovrdval
  Terminator_{1..6} (6 alike) : Terminator
  True_VHAL_SRRBSDWarnL_enum : Constant  Value=TRUE  OutDataTypeStr=boolean
  True_VHAL_SRRBSDWarnR_enum : Constant  Value=TRUE  OutDataTypeStr=boolean
  True_VHAL_SRRODASoundL_flg : Constant  Value=TRUE  OutDataTypeStr=boolean
  True_VHAL_SRRODASoundR_flg : Constant  Value=TRUE  OutDataTypeStr=boolean
  True_VHAL_SRRODAWarnL_enum : Constant  Value=TRUE  OutDataTypeStr=boolean
  True_VHAL_SRRODAWarnR_enum : Constant  Value=TRUE  OutDataTypeStr=boolean
  slr1_{1..6} (6 alike) : BusSelector  OutputSignals=VINP_CANMsgValidSRR1_flg
  slr_VHAL_SRRBSDWarnL_enum : BusSelector  OutputSignals=VHAL_SRRBSDWarnL_enum
  slr_VHAL_SRRBSDWarnR_enum : BusSelector  OutputSignals=VHAL_SRRBSDWarnR_enum
  slr_VHAL_SRRODASoundL_flg : BusSelector  OutputSignals=VHAL_SRRODASoundL_flg
  slr_VHAL_SRRODASoundR_flg : BusSelector  OutputSignals=VHAL_SRRODASoundR_flg
  slr_VHAL_SRRODAWarnL_enum : BusSelector  OutputSignals=VHAL_SRRODAWarnL_enum
  slr_VHAL_SRRODAWarnR_enum : BusSelector  OutputSignals=VHAL_SRRODAWarnR_enum
  VINP_SRRBSDWarnL_enum : Outport
  VINP_SRRBSDWarnR_enum : Outport  Port=2
  VINP_SRRODASoundL_flg : Outport  Port=3
  VINP_SRRODASoundR_flg : Outport  Port=4
  VINP_SRRODAWarnL_enum : Outport  Port=5
  VINP_SRRODAWarnR_enum : Outport  Port=6
  wires:
  BHAL_outputs/1 -> [BHAL_outputs]
  inp_CanValid_bus/1 -> [inp_CanValid_bus]
  [BHAL_outputs] -> slr_VHAL_SRRBSDWarnL_enum/1
  slr_VHAL_SRRBSDWarnL_enum/1 -> SRRBSDWarnL/1  "<VHAL_SRRBSDWarnL_enum>"
  True_VHAL_SRRBSDWarnL_enum/1 -> SRRBSDWarnL/2
  [inp_CanValid_bus] -> slr1_1/1
  slr1_1/1 -> SRRBSDWarnL/3  "<VINP_CANMsgValidSRR1_flg>"
  SRRBSDWarnL/1 -> VINP_SRRBSDWarnL_enum/1  "VINP_SRRBSDWarnL_enum"
  SRRBSDWarnL/2 -> Terminator_1/1
  [BHAL_outputs] -> slr_VHAL_SRRBSDWarnR_enum/1
  slr_VHAL_SRRBSDWarnR_enum/1 -> SRRBSDWarnR/1  "<VHAL_SRRBSDWarnR_enum>"
  True_VHAL_SRRBSDWarnR_enum/1 -> SRRBSDWarnR/2
  [inp_CanValid_bus] -> slr1_2/1
  slr1_2/1 -> SRRBSDWarnR/3  "<VINP_CANMsgValidSRR1_flg>"
  SRRBSDWarnR/1 -> VINP_SRRBSDWarnR_enum/1  "VINP_SRRBSDWarnR_enum"
  SRRBSDWarnR/2 -> Terminator_2/1
  [BHAL_outputs] -> slr_VHAL_SRRODASoundL_flg/1
  slr_VHAL_SRRODASoundL_flg/1 -> SRRODASoundL/1  "<VHAL_SRRODASoundL_flg>"
  True_VHAL_SRRODASoundL_flg/1 -> SRRODASoundL/2
  [inp_CanValid_bus] -> slr1_3/1
  slr1_3/1 -> SRRODASoundL/3  "<VINP_CANMsgValidSRR1_flg>"
  SRRODASoundL/1 -> VINP_SRRODASoundL_flg/1  "VINP_SRRODASoundL_flg"
  SRRODASoundL/2 -> Terminator_3/1
  [BHAL_outputs] -> slr_VHAL_SRRODASoundR_flg/1
  slr_VHAL_SRRODASoundR_flg/1 -> SRRODASoundR/1  "<VHAL_SRRODASoundR_flg>"
  True_VHAL_SRRODASoundR_flg/1 -> SRRODASoundR/2
  [inp_CanValid_bus] -> slr1_4/1
  slr1_4/1 -> SRRODASoundR/3  "<VINP_CANMsgValidSRR1_flg>"
  SRRODASoundR/1 -> VINP_SRRODASoundR_flg/1  "VINP_SRRODASoundR_flg"
  SRRODASoundR/2 -> Terminator_4/1
  [BHAL_outputs] -> slr_VHAL_SRRODAWarnL_enum/1
  slr_VHAL_SRRODAWarnL_enum/1 -> SRRODAWarnL/1  "<VHAL_SRRODAWarnL_enum>"
  True_VHAL_SRRODAWarnL_enum/1 -> SRRODAWarnL/2
  [inp_CanValid_bus] -> slr1_5/1
  slr1_5/1 -> SRRODAWarnL/3  "<VINP_CANMsgValidSRR1_flg>"
  SRRODAWarnL/1 -> VINP_SRRODAWarnL_enum/1  "VINP_SRRODAWarnL_enum"
  SRRODAWarnL/2 -> Terminator_5/1
  [BHAL_outputs] -> slr_VHAL_SRRODAWarnR_enum/1
  slr_VHAL_SRRODAWarnR_enum/1 -> SRRODAWarnR/1  "<VHAL_SRRODAWarnR_enum>"
  True_VHAL_SRRODAWarnR_enum/1 -> SRRODAWarnR/2
  [inp_CanValid_bus] -> slr1_6/1
  slr1_6/1 -> SRRODAWarnR/3  "<VINP_CANMsgValidSRR1_flg>"
  SRRODAWarnR/1 -> VINP_SRRODAWarnR_enum/1  "VINP_SRRODAWarnR_enum"
  SRRODAWarnR/2 -> Terminator_6/1
